simulink model "Daszboard_wersjafinalowa"  (R2015a)
settings: Solver=ode23tb  StartTime=0.0  StopTime=inf
libraries: powerlib x24, powerlib_meascontrol x4
settings Model: Creator=frfr  LastModifiedBy=frfr

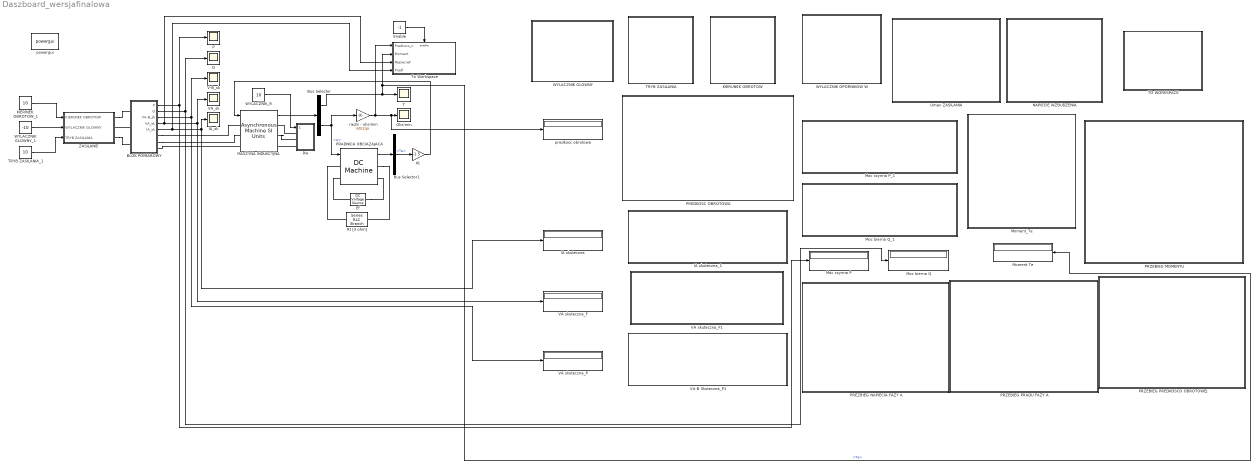
== system Daszboard_wersjafinalowa ==
  BLOK POMIAROWY : Subsystem
  Bus Selector : BusSelector  OutputSignals=Te,w
  Bus Selector1 : BusSelector  OutputSignals=Te
  Ef : powerlib/Electrical Sources/DC Voltage Source  Description=source block  Amplitude=0  Measurements=None
      settings: AttributesFormatString=\n
  Enable : Constant  Value=-1
  IA skuteczna : Display
  IA skuteczna_1 : Subsystem  DialogController=hmiCreateDDGDialog  IsWebBlock=on  mask(MathWorksWebBlock){webBlockId=323fd671-1b8d-4a54-91bf-b9ca35ea488f, webBlockType=lineargauge, ShowInLibBrowser=on, ShowInitialText=on, HMISrcModelName=Daszboard_wersjafinalowa}
      mask prompts: webBlockId "WebBlock Id"; webBlockType "WebBlock Type"; HMISrcModelName "Source Model"
      mask Help: helpview([docroot '/mapfiles/simulink.map'], 'hmi_linear_gauge')
      mask Display:
      | if strcmp(get_param(bdroot(gcb),'BlockDiagramType'), 'library')
      |     image([(matlabroot) '/toolbox/simulink/hmi/icons/LinearGauge.png']);
      | end
  IA_sk : Scope
      settings: SaveName=ScopeData4
  KIERINEK OBROTOW_1 : Constant  Value=10
  KIERUNEK OBROTOW : Subsystem  DialogController=hmiCreateDDGDialog  IsWebBlock=on  mask(MathWorksWebBlock){webBlockId=74e09da8-2fe0-4ee9-b8cf-ca0001514b1b, webBlockType=discreteknob, ShowInLibBrowser=on, ShowInitialText=on, HMISrcModelName=Daszboard_wersjafinalowa}
      mask prompts: webBlockId "WebBlock Id"; webBlockType "WebBlock Type"; HMISrcModelName "Source Model"
      mask Help: helpview([docroot '/mapfiles/simulink.map'], 'hmi_rotary_switch')
      mask Display:
      | model = bdroot(gcb);
      | if strcmp(get_param(model,'BlockDiagramType'), 'library')
      |     image([(matlabroot) '/toolbox/simulink/hmi/icons/DiscreteKnob.png']);
      | end
  Kt : Gain  Gain=-1.5
  MASZYNA INDUKCYJNA : powerlib/Machines/Asynchronous Machine SI Units  RotorType=Wound  PresetModel=No  MechanicalLoad=Torque Tm  ShowDetailedParameters=on  ReferenceFrame=Stationary  Units=SI  MeasurementBus=on  NominalParameters=[ 3000, 380, 50 ]  Stator="[ 1.2  0.0106 ]"  Rotor="[ 1.91  0.0106 ]"  Cage1=[ 0.022 0.226/377]  Cage2=[ 0.022 0.226/377]  Lm=0.2389  Mechanical="[ 0.55  8.25e-3 2]"  PolePairs=2  InitialConditions="[ 1,0   0,0,0   0,0,0 ]"  SimulateSaturation=off  Saturation=[14.03593122, 27.81365428, 53.79336849, 72.68890987, 97.98006896, 148.6815601, 215.7428561, 302.9841135, 428.7778367 ; 230, 322, 414, 460, 506, 552, 598, 644, 690]  LoadFlowParameters=0  TsPowergui=0  TsBlock=-1  IterativeModel=Trapezoidal non iterative  Pmec=0
  Moc bierna Q : Display
  Moc bierna Q_1 : Subsystem  DialogController=hmiCreateDDGDialog  IsWebBlock=on  mask(MathWorksWebBlock){webBlockId=d206d544-67fe-4a45-b1c3-8c19eb73d525, webBlockType=lineargauge, ShowInLibBrowser=on, ShowInitialText=on, HMISrcModelName=Daszboard_wersjafinalowa}
      mask prompts: webBlockId "WebBlock Id"; webBlockType "WebBlock Type"; HMISrcModelName "Source Model"
      mask Help: helpview([docroot '/mapfiles/simulink.map'], 'hmi_linear_gauge')
      mask Display:
      | if strcmp(get_param(bdroot(gcb),'BlockDiagramType'), 'library')
      |     image([(matlabroot) '/toolbox/simulink/hmi/icons/LinearGauge.png']);
      | end
  Moc czynna P : Display
  Moc czynna P_1 : Subsystem  DialogController=hmiCreateDDGDialog  IsWebBlock=on  mask(MathWorksWebBlock){webBlockId=da4f0fbb-935e-4206-9858-fa754842695f, webBlockType=lineargauge, ShowInLibBrowser=on, ShowInitialText=on, HMISrcModelName=Daszboard_wersjafinalowa}
      mask prompts: webBlockId "WebBlock Id"; webBlockType "WebBlock Type"; HMISrcModelName "Source Model"
      mask Help: helpview([docroot '/mapfiles/simulink.map'], 'hmi_linear_gauge')
      mask Display:
      | if strcmp(get_param(bdroot(gcb),'BlockDiagramType'), 'library')
      |     image([(matlabroot) '/toolbox/simulink/hmi/icons/LinearGauge.png']);
      | end
  Moment Te : Display
  Moment_Te : Subsystem  DialogController=hmiCreateDDGDialog  IsWebBlock=on  mask(MathWorksWebBlock){webBlockId=04dc1047-4de5-412a-a5ac-0cde95f85203, webBlockType=ninetydegreegauge, ShowInLibBrowser=on, ShowInitialText=on, HMISrcModelName=Daszboard_wersjafinalowa}
      mask prompts: webBlockId "WebBlock Id"; webBlockType "WebBlock Type"; HMISrcModelName "Source Model"
      mask Help: helpview([docroot '/mapfiles/simulink.map'], 'hmi_quarter_gauge')
      mask Display:
      | if strcmp(get_param(bdroot(gcb),'BlockDiagramType'), 'library')
      |     image([(matlabroot) '/toolbox/simulink/hmi/icons/NinetyDegreeGauge.png']);
      | end
  NAPIECIE WZBUDZENIA : Subsystem  DialogController=hmiCreateDDGDialog  IsWebBlock=on  mask(MathWorksWebBlock){webBlockId=a9afdf0c-aa0b-46d0-bd09-0b17b9f2618e, webBlockType=continuousknob, ShowInLibBrowser=on, ShowInitialText=on, HMISrcModelName=Daszboard_wersjafinalowa}
      mask prompts: webBlockId "WebBlock Id"; webBlockType "WebBlock Type"; HMISrcModelName "Source Model"
      mask Help: helpview([docroot '/mapfiles/simulink.map'], 'hmi_knob')
      mask Display:
      | if strcmp(get_param(bdroot(gcb),'BlockDiagramType'), 'library')
      |     image([(matlabroot) '/toolbox/simulink/hmi/icons/ContinuousKnob.png']);
      | end
  Obr/min : Scope
      settings: YMin=1493.64  YMax=1493.66
  P : Scope
      settings: TimeRange=0.1315942956302907  YMin=1454.8675  YMax=1470.2225
  PRADNICA OBCIAZAJACA : powerlib/Machines/DC Machine  PresetModel=No  MechanicalLoad=Speed w  FieldType=Wound  ShowDetailedParameters=on  MeasurementBus=on  RLa=[2.5 10.4e-3]  RLf=[179 4.1]  Laf=1.236  MachineConstant=Torque constant (N.m/A)  Ke=1.8  Kt=1.8  J=0.02215  Bm=0.002953  Tf=0.5161  w0=1  Ifinit=1  TsPowergui=0  TsBlock=-1
      settings: AttributesFormatString=\n
  PREDKOSC OBROTOWA : Subsystem  DialogController=hmiCreateDDGDialog  IsWebBlock=on  mask(MathWorksWebBlock){webBlockId=1c3e14ac-4c66-4639-8a64-98b182c76d16, webBlockType=semicirculargauge, ShowInLibBrowser=on, ShowInitialText=on, HMISrcModelName=Daszboard_wersjafinalowa}
      mask prompts: webBlockId "WebBlock Id"; webBlockType "WebBlock Type"; HMISrcModelName "Source Model"
      mask Help: helpview([docroot '/mapfiles/simulink.map'], 'hmi_half_gauge')
      mask Display:
      | if strcmp(get_param(bdroot(gcb),'BlockDiagramType'), 'library')
      |     image([(matlabroot) '/toolbox/simulink/hmi/icons/SemicircularGauge.png']);
      | end
  PREZBIEG NAPIECIA FAZY A : Subsystem  DialogController=hmiCreateDDGDialog  IsWebBlock=on  mask(MathWorksWebBlock){webBlockId=8117955c-1b2a-43ec-a9b3-c542121958b4, webBlockType=sdiscope, ShowInitialText=on, HMISrcModelName=Daszboard_wersjafinalowa}
      mask prompts: webBlockId "WebBlock Id"; webBlockType "WebBlock Type"; HMISrcModelName "Source Model"
      mask Help: helpview([docroot '/mapfiles/simulink.map'], 'hmi_scope')
      mask Display:
      | if strcmp(get_param(bdroot(gcb),'BlockDiagramType'), 'library')
      |     image([(matlabroot) '/toolbox/simulink/hmi/icons/DashboardScope.png']);
      | end
  "PRZEBIEG MOMENTU " : Subsystem  DialogController=hmiCreateDDGDialog  IsWebBlock=on  mask(MathWorksWebBlock){webBlockId=f0e19d26-15a5-43b0-a316-7db70fd56646, webBlockType=sdiscope, ShowInitialText=on, HMISrcModelName=Daszboard_wersjafinalowa}
      mask prompts: webBlockId "WebBlock Id"; webBlockType "WebBlock Type"; HMISrcModelName "Source Model"
      mask Help: helpview([docroot '/mapfiles/simulink.map'], 'hmi_scope')
      mask Display:
      | if strcmp(get_param(bdroot(gcb),'BlockDiagramType'), 'library')
      |     image([(matlabroot) '/toolbox/simulink/hmi/icons/DashboardScope.png']);
      | end
  PRZEBIEG PRADU FAZY A : Subsystem  DialogController=hmiCreateDDGDialog  IsWebBlock=on  mask(MathWorksWebBlock){webBlockId=2235004b-d620-4884-b0c6-80f2cd764103, webBlockType=sdiscope, ShowInitialText=on, HMISrcModelName=Daszboard_wersjafinalowa}
      mask prompts: webBlockId "WebBlock Id"; webBlockType "WebBlock Type"; HMISrcModelName "Source Model"
      mask Help: helpview([docroot '/mapfiles/simulink.map'], 'hmi_scope')
      mask Display:
      | if strcmp(get_param(bdroot(gcb),'BlockDiagramType'), 'library')
      |     image([(matlabroot) '/toolbox/simulink/hmi/icons/DashboardScope.png']);
      | end
  PRZEBIEG PREDKOSCO OBROTOWEJ : Subsystem  DialogController=hmiCreateDDGDialog  IsWebBlock=on  mask(MathWorksWebBlock){webBlockId=e683c928-a36a-457c-a764-559816b3a93b, webBlockType=sdiscope, ShowInitialText=on, HMISrcModelName=Daszboard_wersjafinalowa}
      mask prompts: webBlockId "WebBlock Id"; webBlockType "WebBlock Type"; HMISrcModelName "Source Model"
      mask Help: helpview([docroot '/mapfiles/simulink.map'], 'hmi_scope')
      mask Display:
      | if strcmp(get_param(bdroot(gcb),'BlockDiagramType'), 'library')
      |     image([(matlabroot) '/toolbox/simulink/hmi/icons/DashboardScope.png']);
      | end
  Q : Scope
      settings: TimeRange=0.1315942956302907  YMin=1454.8675  YMax=1470.2225  SaveName=ScopeData2
  Rt [3 ohm] : powerlib/Elements/Series RLC Branch  LConnTagsString=__new0  RConnTagsString=__new0  BranchType=R  Resistance=3  Inductance=[]  SetiL0=off  InitialCurrent=0  Capacitance=[]  Setx0=off  InitialVoltage=0  Measurements=None
  Rw : Subsystem
  T : Scope
      settings: SaveName=ScopeData6
  TO WORKSPACE : Subsystem  DialogController=hmiCreateDDGDialog  IsWebBlock=on  mask(MathWorksWebBlock){webBlockId=0fe70ad4-f754-4ac4-96eb-19008607a5f1, webBlockType=discreteknob, ShowInLibBrowser=on, ShowInitialText=on, HMISrcModelName=Daszboard_wersjafinalowa}
      mask prompts: webBlockId "WebBlock Id"; webBlockType "WebBlock Type"; HMISrcModelName "Source Model"
      mask Help: helpview([docroot '/mapfiles/simulink.map'], 'hmi_rotary_switch')
      mask Display:
      | model = bdroot(gcb);
      | if strcmp(get_param(model,'BlockDiagramType'), 'library')
      |     image([(matlabroot) '/toolbox/simulink/hmi/icons/DiscreteKnob.png']);
      | end
  TRYB ZASILANIA : Subsystem  DialogController=hmiCreateDDGDialog  IsWebBlock=on  mask(MathWorksWebBlock){webBlockId=b7b93038-d2fd-4199-8cae-1167181d4641, webBlockType=discreteknob, ShowInLibBrowser=on, ShowInitialText=on, HMISrcModelName=Daszboard_wersjafinalowa}
      mask prompts: webBlockId "WebBlock Id"; webBlockType "WebBlock Type"; HMISrcModelName "Source Model"
      mask Help: helpview([docroot '/mapfiles/simulink.map'], 'hmi_rotary_switch')
      mask Display:
      | model = bdroot(gcb);
      | if strcmp(get_param(model,'BlockDiagramType'), 'library')
      |     image([(matlabroot) '/toolbox/simulink/hmi/icons/DiscreteKnob.png']);
      | end
  TRYB ZASILANIA_1 : Constant  Value=10
  To Workspace : Subsystem
  Umax ZASILANIA : Subsystem  DialogController=hmiCreateDDGDialog  IsWebBlock=on  mask(MathWorksWebBlock){webBlockId=e89c85af-a0c4-44e9-93ad-e130ae210edb, webBlockType=continuousknob, ShowInLibBrowser=on, ShowInitialText=on, HMISrcModelName=Daszboard_wersjafinalowa}
      mask prompts: webBlockId "WebBlock Id"; webBlockType "WebBlock Type"; HMISrcModelName "Source Model"
      mask Help: helpview([docroot '/mapfiles/simulink.map'], 'hmi_knob')
      mask Display:
      | if strcmp(get_param(bdroot(gcb),'BlockDiagramType'), 'library')
      |     image([(matlabroot) '/toolbox/simulink/hmi/icons/ContinuousKnob.png']);
      | end
  V-B_sk : Scope
      settings: SaveName=ScopeData5
  VA skuteczna_F : Display
  VA skuteczna_F1 : Subsystem  DialogController=hmiCreateDDGDialog  IsWebBlock=on  mask(MathWorksWebBlock){webBlockId=11b7919e-c396-40f1-9f33-8d2287d354b0, webBlockType=lineargauge, ShowInLibBrowser=on, ShowInitialText=on, HMISrcModelName=Daszboard_wersjafinalowa}
      mask prompts: webBlockId "WebBlock Id"; webBlockType "WebBlock Type"; HMISrcModelName "Source Model"
      mask Help: helpview([docroot '/mapfiles/simulink.map'], 'hmi_linear_gauge')
      mask Display:
      | if strcmp(get_param(bdroot(gcb),'BlockDiagramType'), 'library')
      |     image([(matlabroot) '/toolbox/simulink/hmi/icons/LinearGauge.png']);
      | end
  VA skuteczna_P : Display
  VA-B Skuteczna_P1 : Subsystem  DialogController=hmiCreateDDGDialog  IsWebBlock=on  mask(MathWorksWebBlock){webBlockId=98d927ca-68bd-43be-a92f-ea2dc9df2090, webBlockType=lineargauge, ShowInLibBrowser=on, ShowInitialText=on, HMISrcModelName=Daszboard_wersjafinalowa}
      mask prompts: webBlockId "WebBlock Id"; webBlockType "WebBlock Type"; HMISrcModelName "Source Model"
      mask Help: helpview([docroot '/mapfiles/simulink.map'], 'hmi_linear_gauge')
      mask Display:
      | if strcmp(get_param(bdroot(gcb),'BlockDiagramType'), 'library')
      |     image([(matlabroot) '/toolbox/simulink/hmi/icons/LinearGauge.png']);
      | end
  VA_sk : Scope
      settings: SaveName=ScopeData3
  WYLACZNIK GLOWNY : Subsystem  DialogController=hmiCreateDDGDialog  IsWebBlock=on  mask(MathWorksWebBlock){webBlockId=441d33e1-ff37-4173-8aa4-66414e3e80de, webBlockType=discreteknob, ShowInLibBrowser=on, ShowInitialText=on, HMISrcModelName=Daszboard_wersjafinalowa}
      mask prompts: webBlockId "WebBlock Id"; webBlockType "WebBlock Type"; HMISrcModelName "Source Model"
      mask Help: helpview([docroot '/mapfiles/simulink.map'], 'hmi_rotary_switch')
      mask Display:
      | model = bdroot(gcb);
      | if strcmp(get_param(model,'BlockDiagramType'), 'library')
      |     image([(matlabroot) '/toolbox/simulink/hmi/icons/DiscreteKnob.png']);
      | end
  WYLACZNIK GLOWNY_1 : Constant  Value=-10
  WYLACZNIK OPORNIKOW W : Subsystem  DialogController=hmiCreateDDGDialog  IsWebBlock=on  mask(MathWorksWebBlock){webBlockId=df9eeaec-f071-4d9e-a568-39a1dac7dec5, webBlockType=discreteknob, ShowInLibBrowser=on, ShowInitialText=on, HMISrcModelName=Daszboard_wersjafinalowa}
      mask prompts: webBlockId "WebBlock Id"; webBlockType "WebBlock Type"; HMISrcModelName "Source Model"
      mask Help: helpview([docroot '/mapfiles/simulink.map'], 'hmi_rotary_switch')
      mask Display:
      | model = bdroot(gcb);
      | if strcmp(get_param(model,'BlockDiagramType'), 'library')
      |     image([(matlabroot) '/toolbox/simulink/hmi/icons/DiscreteKnob.png']);
      | end
  WYLACZNIK_R : Constant  Value=10
  ZASILANIE : Subsystem
  powergui : powerlib/powergui  Priority=1  SimulationMode=Continuous  SolverType=Tustin/Backward Euler (TBE)  SampleTime=50e-6  frequency=60  SPID=on  DisableSnubberDevices=off  DisableRonSwitches=off  DisableVfSwitches=off  SwTol=0  DisplayEquations=off  Interpol=off  methode=off  Ts=100  FunctionMessages=off  echomessages=off  HookPort=off  EnableUseOfTLC=off  x0status=blocks  frequencyindice=0  Pbase=100e6  ErrMax=1e-4  Iterations=50  UnitsV=kV  UnitsW=MW  buscounter=0  RestoreLinks=warning  ResistiveCurrentMeasurement=off  Frange=[0:2:500]  Ylog=off  Xlog=on  ShowGrid=off  save=off  variable=ZData  structure=0  ZoomFFT=off  StartTime=0.0  cycles=1  DisplayStyle=1  fundamental=60  FreqAxis=off  MaxFrequency=1000  frequencyindicesteady=1  RmsSteady=1  display=off
  predkosc obrotowa : Display
  rad/s - obr/min : Gain  Gain=60/2/pi
  wires:
  Bus Selector/2 -> rad/s - obr/min/1, PRADNICA OBCIAZAJACA/1  "<w>"
  rad/s - obr/min/1 -> predkosc obrotowa/1, Obr/min/1, To Workspace/1(Predkocs_n)
  MASZYNA INDUKCYJNA/1 -> Bus Selector/1
  PRADNICA OBCIAZAJACA/1 -> Bus Selector1/1
  KIERINEK OBROTOW_1/1 -> ZASILANIE/1(KIERUNEK OBROTOW)
  WYLACZNIK GLOWNY_1/1 -> ZASILANIE/2(WYLACZNIK GLOWNY)
  Enable/1 -> To Workspace/Enable
  WYLACZNIK_R/1 -> Rw/1(WylacznikR)
  TRYB ZASILANIA_1/1 -> ZASILANIE/3(TRYB ZASILANIA)
  BLOK POMIAROWY/1(P) -> Moc czynna P/1, P/1
  BLOK POMIAROWY/2(Q) -> Moc bierna Q/1, Q/1
  BLOK POMIAROWY/4(VA_sk) -> VA_sk/1, VA skuteczna_F/1, To Workspace/3(NapiecieF)
  BLOK POMIAROWY/5(IA_sk) -> IA_sk/1, IA skuteczna/1, To Workspace/4(Pradf)
  Bus Selector1/1 -> Kt/1  "<Te>"
  Kt/1 -> MASZYNA INDUKCYJNA/1
  BLOK POMIAROWY/3(VA-B_sk) -> V-B_sk/1, VA skuteczna_P/1
  Bus Selector/1 -> T/1, Moment Te/1, To Workspace/2(Moment)  "<Te>"
  connections:
  PRADNICA OBCIAZAJACA/RConn1 -- Rt [3 ohm]/RConn1
  Ef/RConn1 -- PRADNICA OBCIAZAJACA/LConn2
  Ef/LConn1 -- PRADNICA OBCIAZAJACA/RConn2
  Rt [3 ohm]/LConn1 -- PRADNICA OBCIAZAJACA/LConn1
  Rw/LConn1 -- MASZYNA INDUKCYJNA/RConn1
  MASZYNA INDUKCYJNA/RConn2 -- Rw/LConn2
  Rw/LConn3 -- MASZYNA INDUKCYJNA/RConn3
  ZASILANIE/RConn1 -- BLOK POMIAROWY/LConn1
  BLOK POMIAROWY/RConn1 -- MASZYNA INDUKCYJNA/LConn1
  BLOK POMIAROWY/LConn2 -- ZASILANIE/RConn2
  BLOK POMIAROWY/RConn2 -- MASZYNA INDUKCYJNA/LConn2
  ZASILANIE/RConn3 -- BLOK POMIAROWY/LConn3
  BLOK POMIAROWY/RConn3 -- MASZYNA INDUKCYJNA/LConn3

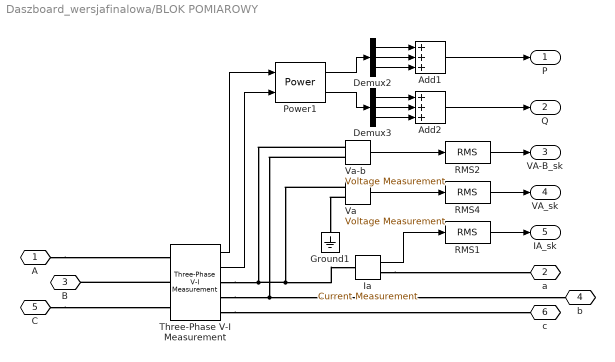
== system Daszboard_wersjafinalowa/BLOK POMIAROWY ==
  Add1 : Sum  Inputs=+++
  Add2 : Sum  Inputs=+++
  Demux2 : Demux  Outputs=3
  Demux3 : Demux  Outputs=3
  Ground1 : powerlib/Elements/Ground  LConnTagsString=a
  Ia : powerlib/Measurements/Current Measurement  PhasorSimulation=off  OutputType=Complex  PSBequivalent=0
  Power1 : powerlib_meascontrol/Measurements/Power  Freq=50  Vinit=[1, 0]  Iinit=[1, 0]  Ts=0
  RMS1 : powerlib_meascontrol/Measurements/RMS  TrueRMS=on  Freq=50  RMSInit=120  Ts=0
  RMS2 : powerlib_meascontrol/Measurements/RMS  TrueRMS=on  Freq=50  RMSInit=120  Ts=0
  RMS4 : powerlib_meascontrol/Measurements/RMS  TrueRMS=on  Freq=50  RMSInit=120  Ts=0
  Three-Phase V-I Measurement : powerlib/Measurements/Three-Phase V-I Measurement  VoltageMeasurement=phase-to-ground  SetLabelV=off  LabelV=Vabc  Vpu=off  VpuLL=off  CurrentMeasurement=yes  SetLabelI=off  LabelI=Iabc  Ipu=off  Pbase=100e6  Vbase=500e3  OutputType=Complex  PhasorSimulation=off  PSBequivalent=0
  "Va " : powerlib/Measurements/Voltage Measurement  PhasorSimulation=off  OutputType=Complex  PSBequivalent=0
  Va-b : powerlib/Measurements/Voltage Measurement  PhasorSimulation=off  OutputType=Complex  PSBequivalent=0
  A : PMIOPort  Port=1  Side=Left
  a : PMIOPort  Port=2  Side=Right
  B : PMIOPort  Port=3  Side=Left
  b : PMIOPort  Port=4  Side=Right
  C : PMIOPort  Port=5  Side=Left
  c : PMIOPort  Port=6  Side=Right
  P : Outport
  Q : Outport  Port=2
  VA-B_sk : Outport  Port=3
  VA_sk : Outport  Port=4
  IA_sk : Outport  Port=5
  wires:
  RMS4/1 -> VA_sk/1
  Demux2/2 -> Add1/2
  Demux3/3 -> Add2/3
  Demux2/1 -> Add1/1
  Demux3/1 -> Add2/1
  Add1/1 -> P/1
  Power1/2 -> Demux3/1
  Demux3/2 -> Add2/2
  Power1/1 -> Demux2/1
  Demux2/3 -> Add1/3
  "Va "/1 -> RMS4/1
  Ia/1 -> RMS1/1
  RMS1/1 -> IA_sk/1
  Add2/1 -> Q/1
  Three-Phase V-I Measurement/1 -> Power1/1
  Three-Phase V-I Measurement/2 -> Power1/2
  Va-b/1 -> RMS2/1
  RMS2/1 -> VA-B_sk/1
  connections:
  Three-Phase V-I Measurement/RConn2 -- b/RConn1 -- Va-b/LConn2
  A/RConn1 -- Three-Phase V-I Measurement/LConn1
  Ia/RConn1 -- a/RConn1
  "Va "/LConn2 -- Ground1/LConn1
  "Va "/LConn1 -- Three-Phase V-I Measurement/RConn1 -- Va-b/LConn1 -- Ia/LConn1
  Three-Phase V-I Measurement/LConn2 -- B/RConn1
  C/RConn1 -- Three-Phase V-I Measurement/LConn3
  Three-Phase V-I Measurement/RConn3 -- c/RConn1

== system Daszboard_wersjafinalowa/IA skuteczna_1 ==

== system Daszboard_wersjafinalowa/KIERUNEK OBROTOW ==

== system Daszboard_wersjafinalowa/Moc bierna Q_1 ==

== system Daszboard_wersjafinalowa/Moc czynna P_1 ==

== system Daszboard_wersjafinalowa/Moment_Te ==

== system Daszboard_wersjafinalowa/NAPIECIE WZBUDZENIA ==

== system Daszboard_wersjafinalowa/PREDKOSC OBROTOWA ==

== system Daszboard_wersjafinalowa/PREZBIEG NAPIECIA FAZY A ==

== system Daszboard_wersjafinalowa/PRZEBIEG MOMENTU  ==

== system Daszboard_wersjafinalowa/PRZEBIEG PRADU FAZY A ==

== system Daszboard_wersjafinalowa/PRZEBIEG PREDKOSCO OBROTOWEJ ==

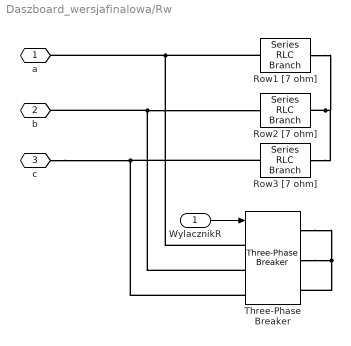
== system Daszboard_wersjafinalowa/Rw ==
  WylacznikR : Inport
  Row1 [7 ohm] : powerlib/Elements/Series RLC Branch  LConnTagsString=__new0  RConnTagsString=__new0  BranchType=R  Resistance=7  Inductance=[]  SetiL0=off  InitialCurrent=0  Capacitance=[]  Setx0=off  InitialVoltage=0  Measurements=None
  Row2 [7 ohm] : powerlib/Elements/Series RLC Branch  LConnTagsString=__new0  RConnTagsString=__new0  BranchType=R  Resistance=7  Inductance=[]  SetiL0=off  InitialCurrent=0  Capacitance=[]  Setx0=off  InitialVoltage=0  Measurements=None
  Row3 [7 ohm] : powerlib/Elements/Series RLC Branch  LConnTagsString=__new0  RConnTagsString=__new0  BranchType=R  Resistance=7  Inductance=[]  SetiL0=off  InitialCurrent=0  Capacitance=[]  Setx0=off  InitialVoltage=0  Measurements=None
  Three-Phase Breaker : powerlib/Elements/Three-Phase Breaker  InitialState=open  SwitchA=on  SwitchB=on  SwitchC=on  SwitchTimes="[1/60  5/60]"  External=on  BreakerResistance=0.01  SnubberResistance=1e6  SnubberCapacitance=inf  Measurements=None
  a : PMIOPort  Port=1  Side=Left
  b : PMIOPort  Port=2  Side=Left
  c : PMIOPort  Port=3  Side=Left
  wires:
  WylacznikR/1 -> Three-Phase Breaker/1
  connections:
  Three-Phase Breaker/LConn1 -- Row1 [7 ohm]/LConn1 -- a/RConn1
  Row2 [7 ohm]/RConn1 -- Row1 [7 ohm]/RConn1 -- Row3 [7 ohm]/RConn1
  Three-Phase Breaker/LConn3 -- c/RConn1 -- Row3 [7 ohm]/LConn1
  Three-Phase Breaker/LConn2 -- b/RConn1 -- Row2 [7 ohm]/LConn1
  Three-Phase Breaker/RConn2 -- Three-Phase Breaker/RConn1 -- Three-Phase Breaker/RConn3

== system Daszboard_wersjafinalowa/TO WORKSPACE ==

== system Daszboard_wersjafinalowa/TRYB ZASILANIA ==

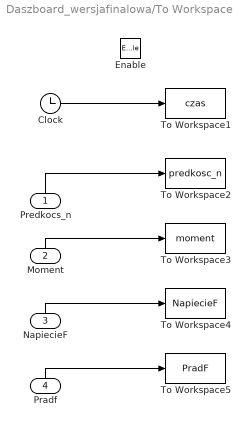
== system Daszboard_wersjafinalowa/To Workspace ==
  Predkocs_n : Inport
  Moment : Inport  Port=2
  NapiecieF : Inport  Port=3
  Pradf : Inport  Port=4
  Enable : EnablePort
  Clock : Clock
  To Workspace1 : ToWorkspace  VariableName=czas  SaveFormat=Timeseries  SampleTime=-1
  To Workspace2 : ToWorkspace  VariableName=predkosc_n  SaveFormat=Timeseries  SampleTime=-1
  To Workspace3 : ToWorkspace  VariableName=moment  SaveFormat=Timeseries  SampleTime=-1
  To Workspace4 : ToWorkspace  VariableName=NapiecieF  SaveFormat=Timeseries  SampleTime=-1
  To Workspace5 : ToWorkspace  VariableName=PradF  SaveFormat=Timeseries  SampleTime=-1
  wires:
  Clock/1 -> To Workspace1/1
  Predkocs_n/1 -> To Workspace2/1
  Moment/1 -> To Workspace3/1
  NapiecieF/1 -> To Workspace4/1
  Pradf/1 -> To Workspace5/1

== system Daszboard_wersjafinalowa/Umax ZASILANIA ==

== system Daszboard_wersjafinalowa/VA skuteczna_F1 ==

== system Daszboard_wersjafinalowa/VA-B Skuteczna_P1 ==

== system Daszboard_wersjafinalowa/WYLACZNIK GLOWNY ==

== system Daszboard_wersjafinalowa/WYLACZNIK OPORNIKOW W ==

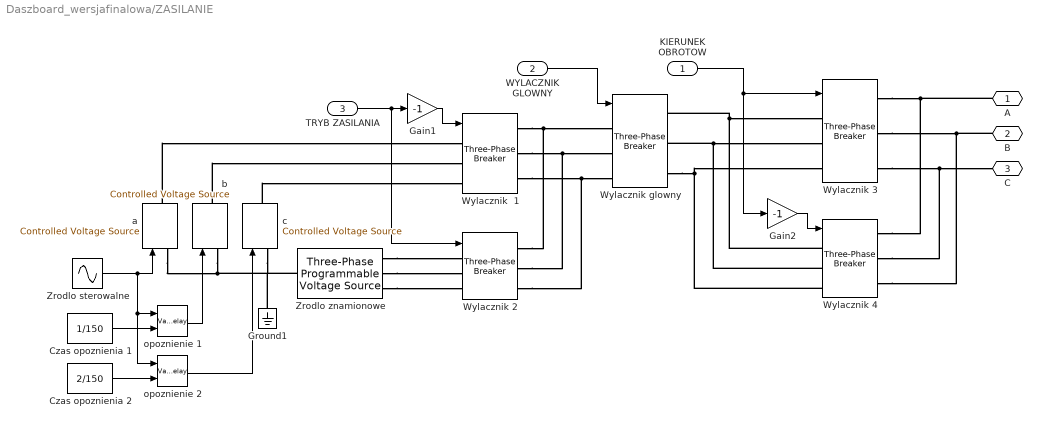
== system Daszboard_wersjafinalowa/ZASILANIE ==
  KIERUNEK OBROTOW : Inport
  WYLACZNIK GLOWNY : Inport  Port=2
  TRYB ZASILANIA : Inport  Port=3
  Czas opoznienia 1 : Constant  Value=1/150
  Czas opoznienia 2 : Constant  Value=2/150
  Gain1 : Gain  Gain=-1
  Gain2 : Gain  Gain=-1
  Ground1 : powerlib/Elements/Ground  LConnTagsString=a
  Wylacznik  1 : powerlib/Elements/Three-Phase Breaker  InitialState=open  SwitchA=on  SwitchB=on  SwitchC=on  SwitchTimes="[1/60  5/60]"  External=on  BreakerResistance=0.01  SnubberResistance=1e6  SnubberCapacitance=inf  Measurements=None
  Wylacznik 2 : powerlib/Elements/Three-Phase Breaker  InitialState=open  SwitchA=on  SwitchB=on  SwitchC=on  SwitchTimes="[1/60  5/60]"  External=on  BreakerResistance=0.01  SnubberResistance=1e6  SnubberCapacitance=inf  Measurements=None
  Wylacznik 3 : powerlib/Elements/Three-Phase Breaker  InitialState=open  SwitchA=on  SwitchB=on  SwitchC=on  SwitchTimes="[1/60  5/60]"  External=on  BreakerResistance=0.01  SnubberResistance=1e6  SnubberCapacitance=inf  Measurements=None
  Wylacznik 4 : powerlib/Elements/Three-Phase Breaker  InitialState=open  SwitchA=on  SwitchB=on  SwitchC=on  SwitchTimes="[1/60  5/60]"  External=on  BreakerResistance=0.01  SnubberResistance=1e6  SnubberCapacitance=inf  Measurements=None
  Wylacznik glowny : powerlib/Elements/Three-Phase Breaker  InitialState=open  SwitchA=on  SwitchB=on  SwitchC=on  SwitchTimes="[1/60  5/60]"  External=on  BreakerResistance=0.01  SnubberResistance=1e6  SnubberCapacitance=inf  Measurements=None
  Zrodlo sterowalne : Sin  Amplitude=0  Frequency=100*pi  SampleTime=0
  Zrodlo znamionowe : powerlib/Electrical Sources/Three-Phase Programmable Voltage Source  PositiveSequence="[380  0 50]"  VariationEntity=None  VariationType=Table of time-amplitude pairs  VariationTypeAlt=Step  VariationStep=0.5  VariationRate=10  VariationMagnitude=0.3  VariationFrequency=2  VariationTiming=[1 2]  VariationPhaseA=off  Amplitudes=[1 0.8 1.2 1.0]  TimeValues=[0 0.1 0.15 0.2]  HarmonicGeneration=off  HarmonicA=[3 0.2 -25 0]  HarmonicB=[2 0.15 35 2]  Timing="[0.05  3]"  BusType=swing  Pref=0  Qref=0  Qmin=-inf  Qmax=inf
  a : powerlib/Electrical Sources/Controlled Voltage Source  Initialize=on  Source_Type=AC  Amplitude=0  Phase=0  Frequency=0  Measurements=None
  b : powerlib/Electrical Sources/Controlled Voltage Source  Initialize=on  Source_Type=AC  Amplitude=0  Phase=120  Frequency=0  Measurements=None
  c : powerlib/Electrical Sources/Controlled Voltage Source  Initialize=on  Source_Type=AC  Amplitude=0  Phase=-120  Frequency=0  Measurements=None
  opoznienie 1 : VariableTransportDelay  MaximumDelay=10
  opoznienie 2 : VariableTransportDelay  MaximumDelay=10
  A : PMIOPort  Port=1  Side=Right
  B : PMIOPort  Port=2  Side=Right
  C : PMIOPort  Port=3  Side=Right
  wires:
  Zrodlo sterowalne/1 -> opoznienie 2/1, opoznienie 1/1, a/1
  Czas opoznienia 1/1 -> opoznienie 1/2
  Czas opoznienia 2/1 -> opoznienie 2/2
  WYLACZNIK GLOWNY/1 -> Wylacznik glowny/1
  KIERUNEK OBROTOW/1 -> Wylacznik 3/1, Gain2/1
  Gain2/1 -> Wylacznik 4/1
  Gain1/1 -> Wylacznik  1/1
  TRYB ZASILANIA/1 -> Wylacznik 2/1, Gain1/1
  opoznienie 1/1 -> b/1
  opoznienie 2/1 -> c/1
  connections:
  a/LConn1 -- b/LConn1 -- c/LConn1 -- Ground1/LConn1 -- Zrodlo znamionowe/LConn1
  Wylacznik 4/LConn2 -- Wylacznik 3/LConn2 -- Wylacznik glowny/RConn2
  Wylacznik 4/LConn1 -- Wylacznik 3/LConn1 -- Wylacznik glowny/RConn1
  Wylacznik 4/LConn3 -- Wylacznik 3/LConn3 -- Wylacznik glowny/RConn3
  Wylacznik 4/RConn3 -- B/RConn1 -- Wylacznik 3/RConn2
  Wylacznik 4/RConn1 -- Wylacznik 3/RConn1 -- A/RConn1
  Wylacznik 4/RConn2 -- Wylacznik 3/RConn3 -- C/RConn1
  Zrodlo znamionowe/RConn1 -- Wylacznik 2/LConn1
  Zrodlo znamionowe/RConn2 -- Wylacznik 2/LConn2
  Zrodlo znamionowe/RConn3 -- Wylacznik 2/LConn3
  Wylacznik  1/RConn2 -- Wylacznik 2/RConn2 -- Wylacznik glowny/LConn2
  Wylacznik  1/RConn1 -- Wylacznik 2/RConn1 -- Wylacznik glowny/LConn1
  Wylacznik 2/RConn3 -- Wylacznik  1/RConn3 -- Wylacznik glowny/LConn3
  c/RConn1 -- Wylacznik  1/LConn3
  b/RConn1 -- Wylacznik  1/LConn2
  a/RConn1 -- Wylacznik  1/LConn1
